simulink model "distribution"  (R2015a)
settings: Solver=ode45  StartTime=0  StopTime=1000  RelTol=1e-3
libraries: simulink x1
(part 1 of 2)
settings Model: Creator=tzimi  LastModifiedBy=Tzimisce

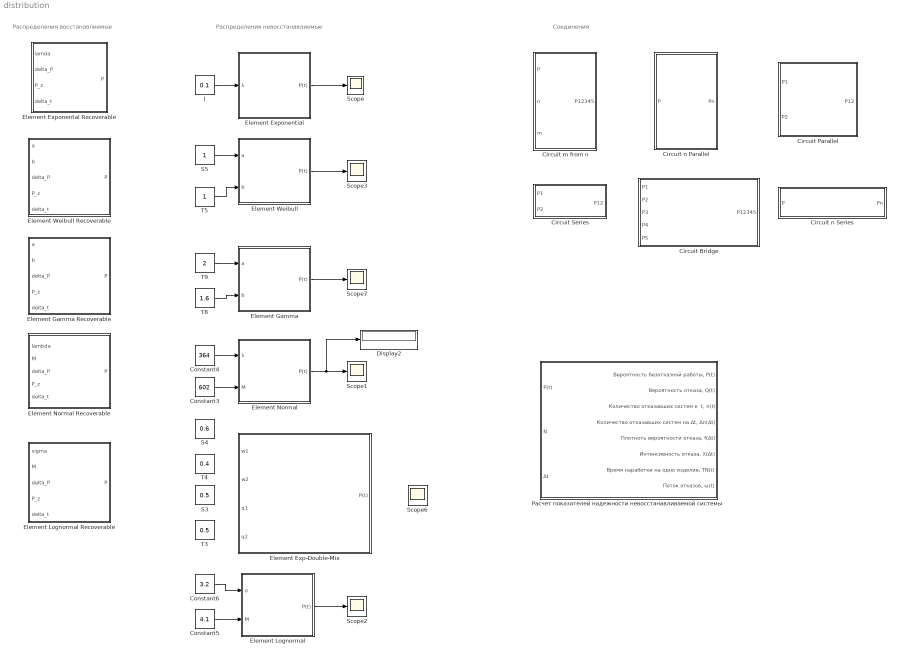
== system distribution ==
  note: Соединения
  note: Распределения невосстанавлиемые
  note: Распределения восстанавлиемые
  Constant3 : Constant  Value=602
  Constant4 : Constant  Value=364
  Constant5 : Constant  Value=4.1
  Constant6 : Constant  Value=3.2
  Display2 : Display
  Element Gamma : Subsystem  mask(Element Gamma){}
      mask help:
      | <p>Возвращает вероятность безотказной работы невосстанавливаемого элемента
      |  по гамма-распределению.</p>
      | <p>Гамма-распределение является результатом смешения большого
      | числа потоков имеющих экспоненциальное распределение.</p>
      | <p>Гамма-распределение используется при оценке надежности объектов, причиной
      | отказа которых является коррозия, вибрация, статическая нагрузка,
      | ошибка персонала и т.д.</p>
      mask Help:
      | <p>Возвращает вероятность безотказной работы невосстанавливаемого элемента
      |  по гамма-распределению.</p>
      | <p>Гамма-распределение используется при оценке надежности объектов, причиной
      | отказа которых является коррозия, вибрация, статическая нагрузка,
      | ошибка персонала и т.д.</p>
      | <p>Входные параметры:</p>
      | <p>a - параметр места гамма-распределения,</p>
      | <p>b - параметр формы гамма-распределения.</p>
      | <p>Выходной параметр P(t) - вероятность безотказной работы элемента.</p>
      mask Display:
      | image('images/png/gamma.png')
      | port_label('input', 1, 'a')
      | port_label('input', 2, 'b')
      | port_label('output', 1, 'P(t)')
  Element Gamma Recoverable : Subsystem  mask(Element Gamma Recoverable){}
      mask help:
      | <p>Возвращает вероятность безотказной работы восстанавливаемого элемента
      | по гамма-распределению.</p>
      | <p>Гамма-распределение является результатом смешения большого
      | числа потоков имеющих экспоненциальное распределение.</p>
      | <p>Гамма-распределение используется при оценке надежности объектов, причиной
      | отказа которых является коррозия, вибрация, статическая нагрузка,
      | ошибка персонала и т.д.</p>
      mask Help:
      | <p>Возвращает вероятность безотказной работы восстанавливаемого элемента
      |  по гамма-распределению.</p>
      | <p>Гамма-распределение используется при оценке надежности объектов, причиной
      | отказа которых является коррозия, вибрация, статическая нагрузка,
      | ошибка персонала и т.д.</p>
      | <p>Входные параметры:</p>
      | <p>a - параметр места гамма-распределения,</p>
      | <p>b - параметр формы гамма-распределения,</p>
      | <p>ΔP - на сколько снижается вероятность безотказной работы после
      | восстановления элемента,</p>
      | <p>Pз - заданная вероятность, после которой проводится восстановление элемента,</p>
      | <p>Δt - время восстановления элемента.</p>
      | <p>Выходной параметр P(t) - вероятность безотказной работы элемента.</p>
      mask Display:
      | image('images/gamma_req.png')
      | port_label('input', 1, 'a')
      | port_label('input', 2, 'b')
      | port_label('input', 3, 'ΔP')
      | port_label('input', 4, 'Pз')
      | port_label('input', 5, 'Δt')
      | port_label('output', 1, 'P(t)')
  Element Exp-Double-Mix : Subsystem  mask(Element Exp-Double-Mix){}
      mask help:
      | <p>Возвращает вероятность безотказной работы двух элементов по экспоненциальному
      | закону распределения.</p>
      | <p>При оценке надежности смеси двух экспоненциальных распределений результатом
      | является поток отказов-восстановлений объектов, составленный из потока отказов
      | с параметром ω1 и потока восстановлений с параметром ω2.</p>
      | <p>Если эти потоки в общем случае не равнодолевые (то есть, не каждый отказ
      | сопровождается полным восстановлением объекта), то необходимо учитывать и
      | доли потоков: q1 и q2 (q1 + q2 = 1).</p>
      mask Help:
      | <p>Возвращает вероятность безотказной работы двух элементов по экспоненциальному
      | закону распределения.</p>
      | <p>Входные параметры:</p>
      | <p>ω1 - поток отказов,</p>
      | <p>ω2 - поток восстановлений,</p>
      | <p>q1 - доля потока отказов,</p>
      | <p>q2 - доля потока восстановления.</p>
      | <p>Выходной параметр P(t) - вероятность безотказной работы элемента.</p>
      mask Display:
      | image('images/png/exp.png')
      | port_label('input', 1, 'ω1')
      | port_label('input', 2, 'ω2')
      | port_label('input', 3, 'q1')
      | port_label('input', 4, 'q2')
      | port_label('output', 1, 'P(t)')
  "Element Exponental Recoverable " : Subsystem  mask(Element Exponental Recoverable){}
      mask help:
      | <p>Возвращает вероятность безотказной работы восстанавливаемого элемента
      | по экспоненциальному закону распределения.</p>
      | <p>Экспоненциальное (или показательное) распределение — абсолютно непрерывное
      | распределение, моделирующее время между двумя последовательными свершениями
      | одного и того же события.</p>
      | <p>Экспоненциальное распределение используют при оценке надежности сложных
      | технических систем, не подверженных износу и старению и в случаях, когда
      | отказы объектов имеют случайный характер.</p>
      mask Help:
      | <p>Возвращает вероятность безотказной работы восстанавливаемого элемента по экспоненциальному
      | закону распределения.</p>
      | <p>Экспоненциальное распределение используют при оценке надежности сложных
      | технических систем, не подверженных износу и старению и в случаях, когда
      | отказы объектов имеют случайный характер.</p>
      | <p>Входные параметры:</p>
      | <p>λ - интенсивность событий в рассматриваемом потоке,</p>
      | <p>ΔP - на сколько снижается вероятность безотказной работы после
      | восстановления элемента,</p>
      | <p>Pз - заданная вероятность, после которой проводится восстановление элемента,</p>
      | <p>Δt - время восстановления элемента.</p>
      | <p>Выходной параметр P(t) - вероятность безотказной работы элемента.</p>
      mask Display:
      | image('images/exp_req.png')
      | port_label('input', 1, 'λ')
      | port_label('input', 2, 'ΔP')
      | port_label('input', 3, 'Pз')
      | port_label('input', 4, 'Δt')
      | port_label('output', 1, 'P(t)')
  Element Exponential : Subsystem  mask(Element Exponential){}
      mask help:
      | <p>Возвращает вероятность безотказной работы невосстанавливаемого элемента
      | по экспоненциальному закону распределения.</p>
      | <p>Экспоненциальное (или показательное) распределение — абсолютно непрерывное
      | распределение, моделирующее время между двумя последовательными свершениями
      | одного и того же события.</p>
      | <p>Экспоненциальное распределение используют при оценке надежности сложных
      | технических систем, не подверженных износу и старению и в случаях, когда
      | отказы объектов имеют случайный характер.</p>
      mask Help:
      | <p>Возвращает вероятность безотказной работы невосстанавливаемого элемента по экспоненциальному
      | закону распределения.</p>
      | <p>Экспоненциальное распределение используют при оценке надежности сложных
      | технических систем, не подверженных износу и старению и в случаях, когда
      | отказы объектов имеют случайный характер.</p>
      | <p>Входной параметр λ - интенсивность событий в рассматриваемом потоке.</p>
      | <p>Выходной параметр P(t) - вероятность безотказной работы элемента.</p>
      mask Display:
      | image('images/png/exp.png')
      | port_label('input', 1, 'λ')
      | port_label('output', 1, 'P(t)')
  "Element Lognormal " : Subsystem  mask(Element Lognormal){}
      mask help:
      | <p>Возвращает вероятность безотказной работы невосстанавливаемого элемента
      | по логнормальному закону распределения.</p>
      | <p>Логнормальное распределение — это двухпараметрическое семейство
      | абсолютно непрерывных распределений. Если случайная величина имеет
      | логнормальное распределение, то её логарифм имеет нормальное распределение.</p>
      | <p>Логнормальное распределение обычно используют при оценке надежности
      | элементов, для которых основной причиной отказа является усталость,
      | обусловленная периодическим многоцикловым (вибрационным) нагружением.</p>
      mask Help:
      | <p>Возвращает вероятность безотказной работы невосстанавливаемого элемента
      | по логнормальному закону распределения.</p>
      | <p>Логнормальное распределение обычно используют при оценке надежности
      | элементов, для которых основной причиной отказа является усталость,
      | обусловленная периодическим многоцикловым (вибрационным) нагружением.</p>
      | <p>Входные параметры:</p>
      | <p>σ - среднее квадратическое отклонение наработки до отказа,</p>
      | <p>М - математическое ожидание наработки до отказа.</p>
      | <p>Выходной параметр P(t) - вероятность безотказной работы элемента.</p>
      mask Display:
      | image('images/png/log_normal.png')
      | port_label('input', 1, 'σ')
      | port_label('input', 2, 'M')
      | port_label('output', 1, 'P(t)')
  Element Lognormal Recoverable : Subsystem  mask(Element Lognormal Recoverable){}
      mask help:
      | <p>Возвращает вероятность безотказной работы восстанавливаемого элемента
      | по логнормальному закону распределения.</p>
      | <p>Логнормальное распределение — это двухпараметрическое семейство
      | абсолютно непрерывных распределений. Если случайная величина имеет
      | логнормальное распределение, то её логарифм имеет нормальное распределение.</p>
      | <p>Логнормальное распределение обычно используют при оценке надежности
      | элементов, для которых основной причиной отказа является усталость,
      | обусловленная периодическим многоцикловым (вибрационным) нагружением.</p>
      mask Help:
      | <p>Возвращает вероятность безотказной работы восстанавливаемого элемента
      | по логнормальному закону распределения.</p>
      | <p>Логнормальное распределение обычно используют при оценке надежности
      | элементов, для которых основной причиной отказа является усталость,
      | обусловленная периодическим многоцикловым (вибрационным) нагружением.</p>
      | <p>Входные параметры:</p>
      | <p>σ - среднее квадратическое отклонение наработки до отказа,</p>
      | <p>М - математическое ожидание наработки до отказа,</p>
      | <p>ΔP - на сколько снижается вероятность безотказной работы после
      | восстановления элемента,</p>
      | <p>Pз - заданная вероятность, после которой проводится восстановление элемента,</p>
      | <p>Δt - время восстановления элемента.</p>
      | <p>Выходной параметр P(t) - вероятность безотказной работы элемента.</p>
      mask Display:
      | image('images/log_normal_req.png')
      | port_label('input', 1, 'σ')
      | port_label('input', 2, 'M')
      | port_label('input', 3, 'ΔP')
      | port_label('input', 4, 'Pз')
      | port_label('input', 5, 'Δt')
      | port_label('output', 1, 'P(t)')
  Element Normal : Subsystem  mask(Element Normal){}
      mask help:
      | <p>Возвращает вероятность безотказной работы невосстанавливаемого
      | элемента по нормальному закону распределения.</p>
      | <p>Нормальное распределение, также называемое распределением Гаусса или
      | Гаусса — Лапласа — распределение вероятностей, которое в одномерном
      | случае задаётся функцией плотности вероятности, совпадающей с функцией
      | Гаусса.</p>
      | <p>Нормальное распределение обычно используют при оценке надежности объектов,
      | основной причиной отказа которых является износ.</p>
      mask Help:
      | <p>Возвращает вероятность безотказной работы невосстанавливаемого
      | элемента по нормальному закону распределения.</p>
      | <p>Нормальное распределение обычно используют при оценке надежности объектов,
      | основной причиной отказа которых является износ.</p>
      | <p>Входные параметры:</p>
      | <p>λ - среднее квадратическое отклонение наработки до отказа,</p>
      | <p>М - математическое ожидание наработки до отказа.</p>
      | <p>Выходной параметр P(t) - вероятность безотказной работы элемента.</p>
      mask Display:
      | image('images/png/normal_nogrid.png')
      | port_label('input', 1, 'λ')
      | port_label('input', 2, 'M')
      | port_label('output', 1, 'P(t)')
  Element Normal Recoverable : Subsystem  mask(Element Normal Recoverable){}
      mask help:
      | <p>Возвращает вероятность безотказной работы восстанавливаемого
      | элемента по нормальному закону распределения.</p>
      | <p>Нормальное распределение, также называемое распределением Гаусса или
      | Гаусса — Лапласа — распределение вероятностей, которое в одномерном
      | случае задаётся функцией плотности вероятности, совпадающей с функцией
      | Гаусса.</p>
      | <p>Нормальное распределение обычно используют при оценке надежности объектов,
      | основной причиной отказа которых является износ.</p>
      mask Help:
      | <p>Возвращает вероятность безотказной работы восстанавливаемого
      | элемента по нормальному закону распределения.</p>
      | <p>Нормальное распределение обычно используют при оценке надежности объектов,
      | основной причиной отказа которых является износ.</p>
      | <p>Входные параметры:</p>
      | <p>λ - среднее квадратическое отклонение наработки до отказа,</p>
      | <p>М - математическое ожидание наработки до отказа,</p>
      | <p>ΔP - на сколько снижается вероятность безотказной работы после
      | восстановления элемента,</p>
      | <p>Pз - заданная вероятность, после которой проводится восстановление элемента,</p>
      | <p>Δt - время восстановления элемента.</p>
      | <p>Выходной параметр P(t) - вероятность безотказной работы элемента.</p>
      mask Display:
      | image('images/normal_nogrid_req.png')
      | port_label('input', 1, 'λ')
      | port_label('input', 2, 'M')
      | port_label('input', 3, 'ΔP')
      | port_label('input', 4, 'Pз')
      | port_label('input', 5, 'Δt')
      | port_label('output', 1, 'P(t)')
  Element Weibull : Subsystem  mask(Element Weibull){}
      mask help:
      | <p>Возвращает вероятность безотказной работы невосстанавливаемого элемента по закону
      | распределения Вейбулла .</p>
      | <p>Распределение Вейбулла — это распределение случайной величины с
      | использованием экспоненты в функциях распределения.</p>
      | <p>Распределение Вейбулла используют для описания закономерностей отказов
      | под действием износа и старения, отказов последовательно соединенных и
      | дублированных элементов. Особенно часто распределение Вейбулла применяют
      | тогда, когда поток отказов не стационарен и интенсивность отказов меняется
      | с течением времени.</p>
      mask Help:
      | <p>Возвращает вероятность безотказной работы невосстанавливаемого элемента по закону
      | распределения Вейбулла .</p>
      | <p>Распределение Вейбулла используют для описания закономерностей отказов
      | под действием износа и старения, отказов последовательно соединенных и
      | дублированных элементов. Особенно часто распределение Вейбулла применяют
      | тогда, когда поток отказов не стационарен и интенсивность отказов меняется
      | с течением времени.</p>
      | <p>Входные параметры:</p>
      | <p>а - параметр места распределения Вейбулла,</p>
      | <p>b - параметр формы распределения Вейбулла.</p>
      | <p>Выходной параметр P(t) - вероятность безотказной работы элемента.</p>
      mask Display:
      | image('images/png/weibull.png')
      | port_label('input', 1, 'a')
      | port_label('input', 2, 'b')
      | port_label('output', 1, 'P(t)')
  Element Weibull Recoverable : Subsystem  mask(Element Weibull Recoverable){}
      mask help:
      | <p>Возвращает вероятность безотказной работы восстанавливаемого элемента по закону
      | распределения Вейбулла .</p>
      | <p>Распределение Вейбулла — это распределение случайной величины с
      | использованием экспоненты в функциях распределения.</p>
      | <p>Распределение Вейбулла используют для описания закономерностей отказов
      | под действием износа и старения, отказов последовательно соединенных и
      | дублированных элементов. Особенно часто распределение Вейбулла применяют
      | тогда, когда поток отказов не стационарен и интенсивность отказов меняется
      | с течением времени.</p>
      mask Help:
      | <p>Возвращает вероятность безотказной работы восстанавливаемого элемента по закону
      | распределения Вейбулла.</p>
      | <p>Распределение Вейбулла используют для описания закономерностей отказов
      | под действием износа и старения, отказов последовательно соединенных и
      | дублированных элементов. Особенно часто распределение Вейбулла применяют
      | тогда, когда поток отказов не стационарен и интенсивность отказов меняется
      | с течением времени.</p>
      | <p>Входные параметры:</p>
      | <p>а - параметр места распределения Вейбулла,</p>
      | <p>b - параметр формы распределения Вейбулла,</p>
      | <p>ΔP - на сколько снижается вероятность безотказной работы после
      | восстановления элемента,</p>
      | <p>Pз - заданная вероятность, после которой проводится восстановление элемента,</p>
      | <p>Δt - время восстановления элемента.</p>
      | <p>Выходной параметр P(t) - вероятность безотказной работы элемента.</p>
      mask Display:
      | image('images/weibull_req.png')
      | port_label('input', 1, 'a')
      | port_label('input', 2, 'b')
      | port_label('input', 3, 'ΔP')
      | port_label('input', 4, 'Pз')
      | port_label('input', 5, 'Δt')
      | port_label('output', 1, 'P(t)')
  S3 : Constant  Value=0.5
  S4 : Constant  Value=0.6
  S5 : Constant
  Scope{,1..3,6..7} (6 alike) : Scope
      Scope settings: YMin=-0.12495  YMax=1.12499
      Scope1 settings: TimeRange=20  YMin=-0.97508  YMax=0.10834
      Scope2 settings: YMin=-2.66158  YMax=1.40684  SaveName=ScopeData2
      Scope3 settings: TimeRange=20  YMin=-0.125  YMax=1.125  SaveName=ScopeData3
      Scope6 settings: YMin=-0.12477  YMax=1.12497  SaveName=ScopeData6
      Scope7 settings: TimeRange=20  YMin=-0.12409  YMax=1.11677  SaveName=ScopeData7
  T3 : Constant  Value=0.5
  T4 : Constant  Value=0.4
  T5 : Constant
  T8 : Constant  Value=1.6
  T9 : Constant  Value=2
  l : Constant  Value=0.1
  Расчет показателей надежности невосстанавливаемой системы : Subsystem  mask(Calculation of reliability indicators of an unrecoverable system.){}
      mask help:
      | <p>Расчет показателей надежности невосстанавливаемой системы.</p>
      | <p>Возвращает показатели надежности невосстанавливаемой системы.</p>
      | <p>Показателями надежности называются количественные характеристики одного
      | или нескольких свойств, составляющих надежность системы.</p>
      mask Help:
      | <p>Возвращает показатели надежности невосстанавливаемой системы.</p>
      | <p>Показателями надежности называются количественные характеристики одного
      | или нескольких свойств, составляющих надежность системы.</p>
      | <p>Входные параметры:</p>
      | <p>P(t)- вероятность безотказной работы элемента,</p>
      | <p>N - количество элементов,</p>
      | <p>Δt - шаг времени.</p>
      | <p>Выходной параметры:</p>
      | <p>P(t)- вероятность безотказной работы элемента,</p>
      | <p>Q(t) - вероятность отказа элемента,</p>
      | <p>n(t) - количество отказавших систем ко времени t,</p>
      | <p>Δn(Δt) - количество отказавших систем на момент времени Δt,</p>
      | <p>f(Δt) - плотноть вероятности отказа,</p>
      | <p>λ(Δt) - интенсивность отказа,</p>
      | <p>TN(t) - время наработки на одно изделие,</p>
      | <p>ω(t) - поток отказов.</p>
      mask Display:
      | port_label('input', 1, 'P(t)')
      | port_label('input', 2, 'N')
      | port_label('input', 3, 'Δt')
      | port_label('output', 1, 'P(t)')
      | port_label('output', 2, 'Q(t)')
      | port_label('output', 3, 'n(t)')
      | port_label('output', 4, 'Δn(Δt)')
      | port_label('output', 5, 'f(Δt)')
      | port_label('output', 6, 'λ(Δt)')
      | port_label('output', 7, 'TN(t)')
      | port_label('output', 8, 'ω(t)')
  Сircuit Bridge : Subsystem  mask(Сircuit Bridge){}
      mask help:
      | <p>Возвращает вероятность безотказной работы пяти элементов, соединенных
      | мостиковой схемой.</p>
      | <p>Мостиковой схемой называется параллельное соединение последовательных
      | цепочек элементов с диагональными элементами, включенными между узлами
      | различных параллельных ветвей.</p>
      | <p>Работоспособность мостиковой схемы зависит не только от количества отказавших
      | элементов, но и от их положения в структурной схеме.</p>
      mask Help:
      | <p>Возвращает вероятность безотказной работы пяти элементов, соединенных
      | мостиковой схемой.</p>
      | <p>Работоспособность мостиковой схемы зависит не только от количества отказавших
      | элементов, но и от их положения в структурной схеме. При одновременном отказе
      | элементов 1 и 4, или 2 и 5, или 2, 3 и 4 и т.д. схема окажется неработоспособной.
      | Но отказ элементов 1 и 5, или 2 и 4, или 1, 3 и 4, или 2, 3 и 5 к отказу
      | системы не приводит.</p>
      | <p>Входные параметры:</p>
      | <p>P1 - вероятность безотказной работы первого элемента,</p>
      | <p>P2 - вероятность безотказной работы второго элемента,</p>
      | <p>P3 - вероятность безотказной работы третьего элемента,</p>
      | <p>P4 - вероятность безотказной работы четвертого элемента,</p>
      | <p>P5 - вероятность безотказной работы пятого элемента.</p>
      | <p>Выходной параметр P(t) - вероятность безотказной работы всех элементов.</p>
      mask Display:
      | image('images\png\bridge.png')
      | port_label('input', 1, 'P1')
      | port_label('input', 2, 'P2')
      | port_label('input', 3, 'P3')
      | port_label('input', 4, 'P4')
      | port_label('input', 5, 'P5')
      | port_label('output', 1, 'P')
  Сircuit Parallel : Subsystem  mask(Сircuit Parallel){}
      mask help:
      | <p>Возвращает вероятность безотказной работы двух параллельно соединенных
      | элементов.</p>
      | <p>В системе с параллельной структурой отказ системы в целом происходит только
      | при отказе всех элементов.</p>
      mask Help:
      | <p>Возвращает вероятность безотказной работы двух параллельно соединенных
      | элементов.</p>
      | <p>Входные параметры:</p>
      | <p>P1 - вероятность безотказной работы первого элемента,</p>
      | <p>P2 - вероятность безотказной работы второго элемента.</p>
      | <p>Выходной параметр P12 - вероятность безотказной работы двух параллельно
      | соединенных элементов.</p>
      mask Display:
      | image('images/png/parallel2.png')
      | port_label('input', 1, 'P1')
      | port_label('input', 2, 'P2')
      | port_label('output', 1, 'P12')
  Сircuit Series : Subsystem  mask(Сircuit Series){}
      mask help:
      | <p>Возвращает вероятность безотказной работы двух последовательно соединенных
      | элементов.</p>
      | <p>В системе с последовательной структурой отказ любого компонента приводит
      | к отказу системы в целом.</p>
      mask Help:
      | <p>Возвращает вероятность безотказной работы двух последовательно соединенных
      | элементов.</p>
      | <p>Входные параметры:</p>
      | <p>P1 - вероятность безотказной работы первого элемента,</p>
      | <p>P2 - вероятность безотказной работы второго элемента.</p>
      | <p>Выходной параметр P12 - вероятность безотказной работы двух последовательно
      | соединенных элементов.</p>
      mask Display:
      | image('images/png/series2.png')
      | port_label('input', 1, 'P1')
      | port_label('input', 2, 'P2')
      | port_label('output', 1, 'P12')
  Сircuit m from n : Subsystem  mask(Сircuit m from n){}
      mask help:
      | <p>Возвращает вероятность того, что в системе, состоящей из n одинаковых
      | (равнонадежных) элементов, безотказно работают ровно m элементов.</p>
      | <p>Система типа “m из n” это вариант системы с параллельным соединением
      | элементов, отказ которой произойдет, если из n элементов, соединенных
      | параллельно, работоспособными окажутся менее m элементов (m < n).</p>
      mask Help:
      | <p>Возвращает вероятность того, что в системе, состоящей из n одинаковых
      | (равнонадежных) элементов, безотказно работают ровно k элементов.</p>
      | <p>Входные параметры:</p>
      | <p>P - вероятность безотказной работы n равнонадежных элементов,</p>
      | <p>n - количество элементов в системе,</p>
      | <p>m - количество элементов, необходимых для работоспособности системы.</p>
      | <p>Выходной параметр Pm - вероятность безотказной работы m элементов системы.</p>
      mask Display:
      | image('images\png\mn.png')
      | port_label('input', 1, 'P')
      | port_label('input', 2, 'n')
      | port_label('input', 3, 'm')
      | port_label('output', 1, 'Pm')
  Сircuit n Parallel : Subsystem  mask(Сircuit n Parallel){}
      mask help:
      | <p>Возвращает вероятность безотказной работы n параллельно соединенных
      | элементов.</p>
      | <p>В системе с параллельной структурой отказ системы в целом происходит только
      | при отказе всех элементов.</p>
      mask Help:
      | <p>Возвращает вероятность безотказной работы n параллельно соединенных
      | элементов.</p>
      | <p>Входной параметр P - массив вероятностей безотказной работы элементов.</p>
      | <p>Выходной параметр Pт - вероятность безотказной работы n параллельно
      | соединенных элементов.</p>
      mask Display:
      | image('images\png\parallel.png')
      | port_label('input', 1, 'P')
      | port_label('output', 1, 'Pn')
  Сircuit n Series : Subsystem  mask(Сircuit n Series){}
      mask help:
      | <p>Возвращает вероятность безотказной работы n последовательно соединенных
      | элементов.</p>
      | <p>В системе с последовательной структурой отказ любого компонента приводит
      | к отказу системы в целом.</p>
      mask Help:
      | <p>Возвращает вероятность безотказной работы n последовательно соединенных
      | элементов.</p>
      | <p>Входной параметр P - массив вероятностей безотказной работы n элементов.</p>
      | <p>Выходной параметр Pn - вероятность безотказной работы n последовательно
      | соединенных элементов.</p>
      mask Display:
      | image('images\png\series.png')
      | port_label('input', 1, 'P')
      | port_label('output', 1, 'Pn')
  wires:
  Constant4/1 -> Element Normal/1("λ ")
  Constant3/1 -> Element Normal/2("M ")
  Element Normal/1(P(t)) -> Display2/1, Scope1/1
  T9/1 -> Element Gamma/1(a)
  T8/1 -> Element Gamma/2(b)
  Element Gamma/1(P(t)) -> Scope7/1
  Element Exponential/1(P(t)) -> Scope/1
  Element Weibull/1(P(t)) -> Scope3/1
  l/1 -> Element Exponential/1("λ ")
  S5/1 -> Element Weibull/1("a ")
  T5/1 -> Element Weibull/2("b ")
  Constant6/1 -> "Element Lognormal "/1("σ ")
  Constant5/1 -> "Element Lognormal "/2("M ")
  "Element Lognormal "/1(P(t)) -> Scope2/1

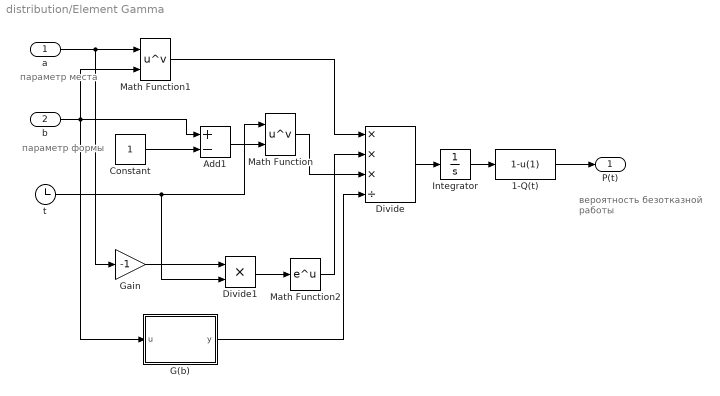
== system distribution/Element Gamma ==
  note: параметр
      | формы
  note: параметр
      | места
  note: вероятность
      | безотказной
      | работы
  a : Inport
  b : Inport  Port=2
  1-Q(t) : Fcn  Expr=1-u(1)
  Add1 : Sum  Inputs=+-
  Constant : Constant
  Divide : Product  Inputs=***/
  Divide1 : Product  Inputs=**
  G(b) : MATLAB Function  TreatAsAtomicUnit=on
  Gain : Gain  Gain=-1
  Integrator : Integrator
  Math Function : Math  Operator=pow  SaturateOnIntegerOverflow=on
  Math Function1 : Math  Operator=pow  SaturateOnIntegerOverflow=on
  Math Function2 : Math  SaturateOnIntegerOverflow=on
  t : Clock
  P(t) : Outport
  wires:
  b/1 -> Add1/1, Math Function1/2, G(b)/1(u)
  Add1/1 -> Math Function/2
  a/1 -> Math Function1/1, Gain/1
  Math Function1/1 -> Divide/1
  Gain/1 -> Divide1/1
  Divide1/1 -> Math Function2/1
  Math Function2/1 -> Divide/2
  Constant/1 -> Add1/2
  1-Q(t)/1 -> P(t)/1
  Divide/1 -> Integrator/1
  Math Function/1 -> Divide/3
  Integrator/1 -> 1-Q(t)/1
  t/1 -> Divide1/2, Math Function/1
  G(b)/1(y) -> Divide/4

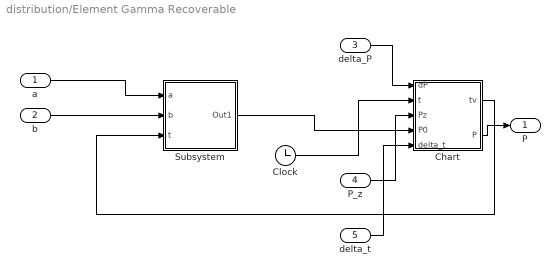
== system distribution/Element Gamma Recoverable ==
  a : Inport
  b : Inport  Port=2
  delta_P : Inport  Port=3
  P_z : Inport  Port=4
  delta_t : Inport  Port=5
  Chart : Stateflow chart  TreatAsAtomicUnit=on
  Clock : Clock
  Subsystem : Subsystem
  P : Outport
  wires:
  Subsystem/1(Out1) -> Chart/4(P0)
  Chart/2(P) -> P/1
  P_z/1 -> Chart/3(Pz)
  delta_P/1 -> Chart/1(dP)
  Clock/1 -> Chart/2(t)
  a/1 -> Subsystem/1(a)
  b/1 -> Subsystem/2(b)
  Chart/1(tv) -> Subsystem/3(t)
  delta_t/1 -> Chart/5(delta_t)

== system distribution/Element Exp-Double-Mix ==
  note: Доля потока
      | восстановления
  note: Доля потока отказов
  note: Параметр поток
      | восстановлений
  note: Параметр поток отказов
  note: вероятность
      | безотказной
      | работы
  "w1 " : Inport
  "w2 " : Inport  Port=2
  "q1 " : Inport  Port=3
  "q2 " : Inport  Port=4
  Mux : Mux  Inputs=5
  f(t) : Fcn  Expr=(u(3)*u(2)*exp((-1)*u(1)*u(5))+u(4)*u(1)*exp((-1)*u(2)*u(5)))/(u(1)*u(4)+u(2)*u(3))
  t : Clock
  P(t) : Outport
  wires:
  "q1 "/1 -> Mux/3
  t/1 -> Mux/5
  "w1 "/1 -> Mux/1
  f(t)/1 -> P(t)/1
  "w2 "/1 -> Mux/2
  "q2 "/1 -> Mux/4
  Mux/1 -> f(t)/1

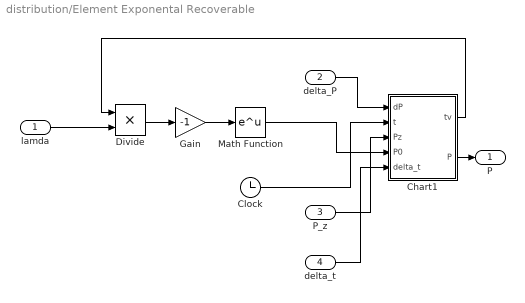
== system distribution/Element Exponental Recoverable  ==
  lamda : Inport
  delta_P : Inport  Port=2
  P_z : Inport  Port=3
  delta_t : Inport  Port=4
  Chart1 : Stateflow chart  TreatAsAtomicUnit=on
  Clock : Clock
  Divide : Product  Inputs=**
  Gain : Gain  Gain=-1
  Math Function : Math  SaturateOnIntegerOverflow=on
  P : Outport
  wires:
  Chart1/2(P) -> P/1
  P_z/1 -> Chart1/3(Pz)
  Math Function/1 -> Chart1/4(P0)
  delta_P/1 -> Chart1/1(dP)
  Chart1/1(tv) -> Divide/1
  Clock/1 -> Chart1/2(t)
  lamda/1 -> Divide/2
  Gain/1 -> Math Function/1
  Divide/1 -> Gain/1
  delta_t/1 -> Chart1/5(delta_t)

== system distribution/Element Exponential ==
  note: интенсивность событий
      | в рассматриваемом потоке
  note: вероятность
      | безотказной
      | работы
  "λ " : Inport
  Divide : Product  Inputs=**
  Gain : Gain  Gain=-1
  Math Function : Math  SaturateOnIntegerOverflow=on
  t : Clock
  P(t) : Outport
  wires:
  Divide/1 -> Gain/1
  t/1 -> Divide/1
  Gain/1 -> Math Function/1
  Math Function/1 -> P(t)/1
  "λ "/1 -> Divide/2

== system distribution/Element Lognormal  ==
  note: среднее квадратическое
      | отклонение наработки
      | до отказа
  note: математическое ожидание
      | наработки до отказа
  note: вероятность
      | безотказной
      | работы
  "σ " : Inport
  "M " : Inport  Port=2
  Fcn1 : Fcn  Expr=1-u(1)
  MATLAB Function : MATLAB Function  TreatAsAtomicUnit=on
  t : Clock
  P(t) : Outport
  wires:
  MATLAB Function/1(y) -> Fcn1/1
  Fcn1/1 -> P(t)/1
  t/1 -> MATLAB Function/1(t)
  "σ "/1 -> MATLAB Function/2(sigma)
  "M "/1 -> MATLAB Function/3(M)

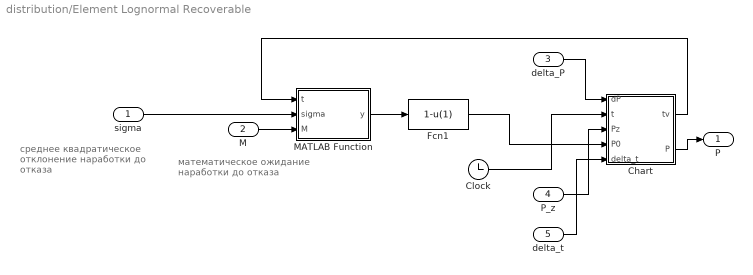
== system distribution/Element Lognormal Recoverable ==
  note: среднее квадратическое
      | отклонение наработки
      | до отказа
  note: математическое ожидание
      | наработки до отказа
  "sigma " : Inport
  "M " : Inport  Port=2
  delta_P : Inport  Port=3
  P_z : Inport  Port=4
  delta_t : Inport  Port=5
  Chart : Stateflow chart  TreatAsAtomicUnit=on
  Clock : Clock
  Fcn1 : Fcn  Expr=1-u(1)
  MATLAB Function : MATLAB Function  TreatAsAtomicUnit=on
  P : Outport
  wires:
  Chart/2(P) -> P/1
  P_z/1 -> Chart/3(Pz)
  delta_P/1 -> Chart/1(dP)
  Clock/1 -> Chart/2(t)
  MATLAB Function/1(y) -> Fcn1/1
  Chart/1(tv) -> MATLAB Function/1(t)
  "sigma "/1 -> MATLAB Function/2(sigma)
  "M "/1 -> MATLAB Function/3(M)
  Fcn1/1 -> Chart/4(P0)
  delta_t/1 -> Chart/5(delta_t)

== system distribution/Element Normal ==
  note: вероятность
      | безотказной
      | работы
  note: математическое ожидание
      | наработки до отказа
  note: среднее квадратическое
      | отклонение наработки
      | до отказа
  "λ " : Inport
  "M " : Inport  Port=2
  1-Q(t)1 : Fcn  Expr=1-u(1)
  MATLAB Function : MATLAB Function  TreatAsAtomicUnit=on
  t : Clock
  P(t) : Outport
  wires:
  MATLAB Function/1(y) -> 1-Q(t)1/1
  "λ "/1 -> MATLAB Function/2(sigma)
  1-Q(t)1/1 -> P(t)/1
  t/1 -> MATLAB Function/1(t)
  "M "/1 -> MATLAB Function/3(M)

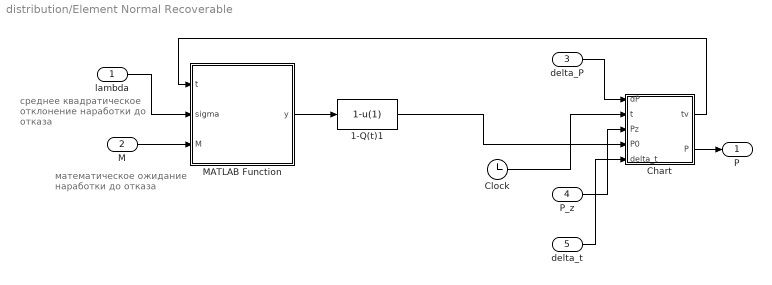
== system distribution/Element Normal Recoverable ==
  note: математическое ожидание
      | наработки до отказа
  note: среднее квадратическое
      | отклонение наработки
      | до отказа
  "lambda " : Inport
  "M " : Inport  Port=2
  delta_P : Inport  Port=3
  P_z : Inport  Port=4
  delta_t : Inport  Port=5
  1-Q(t)1 : Fcn  Expr=1-u(1)
  Chart : Stateflow chart  TreatAsAtomicUnit=on
  Clock : Clock
  MATLAB Function : MATLAB Function  TreatAsAtomicUnit=on
  P : Outport
  wires:
  Clock/1 -> Chart/2(t)
  delta_P/1 -> Chart/1(dP)
  P_z/1 -> Chart/3(Pz)
  Chart/2(P) -> P/1
  1-Q(t)1/1 -> Chart/4(P0)
  MATLAB Function/1(y) -> 1-Q(t)1/1
  "lambda "/1 -> MATLAB Function/2(sigma)
  "M "/1 -> MATLAB Function/3(M)
  Chart/1(tv) -> MATLAB Function/1(t)
  delta_t/1 -> Chart/5(delta_t)

== system distribution/Element Weibull ==
  note: параметр формы
  note: параметр места
  note: вероятность
      | безотказной
      | работы
  "a " : Inport
  "b " : Inport  Port=2
  Mux : Mux  Inputs=3
  f(t) : Fcn  Expr=exp((-1)*u(3)^(u(2))*u(1)^(-1))
  задаваемая наработка : Clock
  P(t) : Outport
  wires:
  "a "/1 -> Mux/1
  f(t)/1 -> P(t)/1
  Mux/1 -> f(t)/1
  задаваемая наработка/1 -> Mux/3
  "b "/1 -> Mux/2

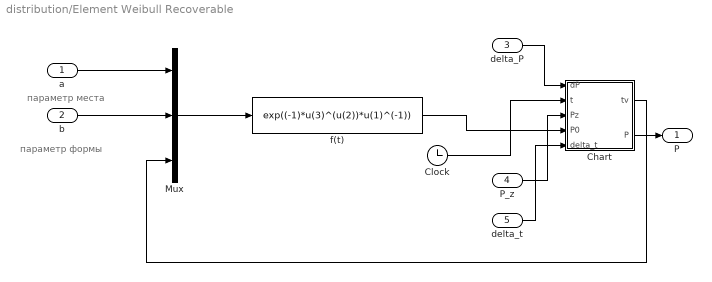
== system distribution/Element Weibull Recoverable ==
  note: параметр формы
  note: параметр места
  "a " : Inport
  "b " : Inport  Port=2
  delta_P : Inport  Port=3
  P_z : Inport  Port=4
  delta_t : Inport  Port=5
  Chart : Stateflow chart  TreatAsAtomicUnit=on
  Clock : Clock
  Mux : Mux  Inputs=3
  f(t) : Fcn  Expr=exp((-1)*u(3)^(u(2))*u(1)^(-1))
  P : Outport
  wires:
  Clock/1 -> Chart/2(t)
  delta_P/1 -> Chart/1(dP)
  P_z/1 -> Chart/3(Pz)
  Chart/2(P) -> P/1
  "a "/1 -> Mux/1
  f(t)/1 -> Chart/4(P0)
  Mux/1 -> f(t)/1
  Chart/1(tv) -> Mux/3
  "b "/1 -> Mux/2
  delta_t/1 -> Chart/5(delta_t)

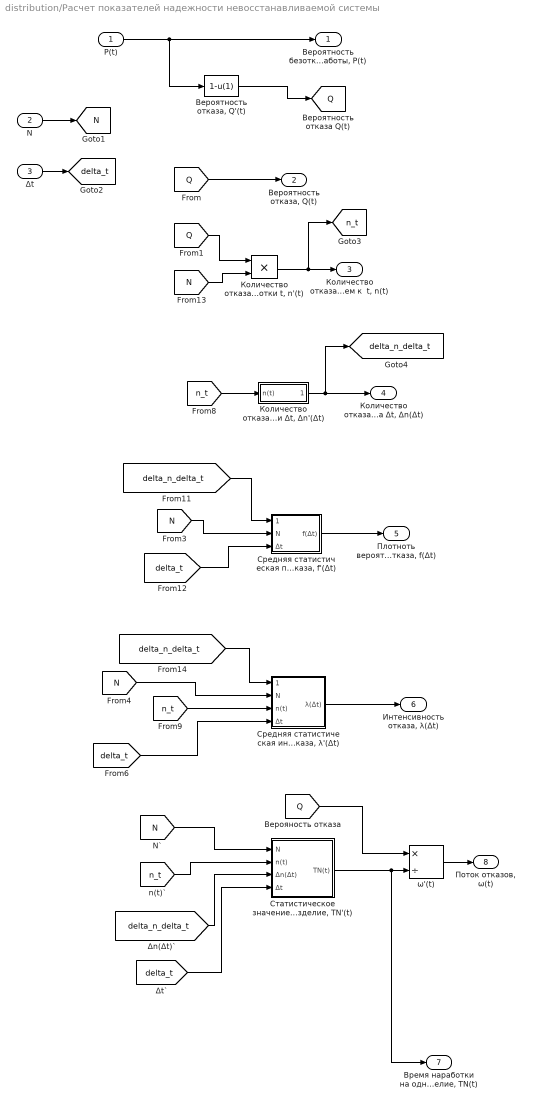
== system distribution/Расчет показателей надежности невосстанавливаемой системы ==
  Р(t) : Inport
  N : Inport  Port=2
  Δt : Inport  Port=3
  ω'(t) : Product  Inputs=*/
  "Вероятность отказа, Q'(t)" : Fcn  Expr=1-u(1)
  "Количество отказавших систем к моменту наработки t, n'(t)" : Product
  "Количество отказавших систем на интервалах наработки Δt, Δn'(Δt)" : Subsystem
  "Средняя статистическая интенсивность отказа, λ'(Δt)" : Subsystem
  "Средняя статистическая плотноть вероятности отказа, f'(Δt)" : Subsystem
  "Статистическое значение среднего времени наработки на одно изделие, TN'(t)" : Subsystem
  "Вероятность безотказной работы, Р(t)" : Outport
  "Вероятность отказа, Q(t)" : Outport  Port=2
  "Количество отказавших систем к  t, n(t)" : Outport  Port=3
  "Количество отказавших систем на Δt, Δn(Δt)" : Outport  Port=4
  "Плотноть вероятности отказа, f(Δt)" : Outport  Port=5
  "Интенсивность отказа, λ(Δt)" : Outport  Port=6
  "Время наработки на одно изделие, TN(t)" : Outport  Port=7
  "Поток отказов, ω(t)" : Outport  Port=8
  tag scope: N=global, Q=global, delta_n_delta_t=global, delta_t=global, n_t=global
  wires:
  [delta_n_delta_t] -> "Статистическое значение среднего времени наработки на одно изделие, TN'(t)"/3(Δn(Δt))
  [delta_n_delta_t] -> "Средняя статистическая интенсивность отказа, λ'(Δt)"/1(Δn(Δt))
  [delta_n_delta_t] -> "Средняя статистическая плотноть вероятности отказа, f'(Δt)"/1(Δn(Δt))
  [N] -> "Количество отказавших систем к моменту наработки t, n'(t)"/2
  [delta_t] -> "Средняя статистическая плотноть вероятности отказа, f'(Δt)"/3(Δt)
  [n_t] -> "Статистическое значение среднего времени наработки на одно изделие, TN'(t)"/2(n(t))
  [n_t] -> "Средняя статистическая интенсивность отказа, λ'(Δt)"/3(n(t))
  [n_t] -> "Количество отказавших систем на интервалах наработки Δt, Δn'(Δt)"/1(n(t))
  [delta_t] -> "Статистическое значение среднего времени наработки на одно изделие, TN'(t)"/4(Δt)
  [delta_t] -> "Средняя статистическая интенсивность отказа, λ'(Δt)"/4(Δt)
  [N] -> "Статистическое значение среднего времени наработки на одно изделие, TN'(t)"/1(N)
  [N] -> "Средняя статистическая интенсивность отказа, λ'(Δt)"/2(N)
  [N] -> "Средняя статистическая плотноть вероятности отказа, f'(Δt)"/2(N)
  [Q] -> ω'(t)/1
  [Q] -> "Количество отказавших систем к моменту наработки t, n'(t)"/1
  [Q] -> "Вероятность отказа, Q(t)"/1
  ω'(t)/1 -> "Поток отказов, ω(t)"/1
  "Вероятность отказа, Q'(t)"/1 -> [Q]
  "Статистическое значение среднего времени наработки на одно изделие, TN'(t)"/1(TN(t)) -> ω'(t)/2, "Время наработки на одно изделие, TN(t)"/1
  N/1 -> [N]
  "Средняя статистическая интенсивность отказа, λ'(Δt)"/1(λ(Δt)) -> "Интенсивность отказа, λ(Δt)"/1
  "Средняя статистическая плотноть вероятности отказа, f'(Δt)"/1(f(Δt)) -> "Плотноть вероятности отказа, f(Δt)"/1
  "Количество отказавших систем к моменту наработки t, n'(t)"/1 -> "Количество отказавших систем к  t, n(t)"/1, [n_t]
  "Количество отказавших систем на интервалах наработки Δt, Δn'(Δt)"/1(Δn(Δt)) -> "Количество отказавших систем на Δt, Δn(Δt)"/1, [delta_n_delta_t]
  Δt/1 -> [delta_t]
  Р(t)/1 -> "Вероятность безотказной работы, Р(t)"/1, "Вероятность отказа, Q'(t)"/1

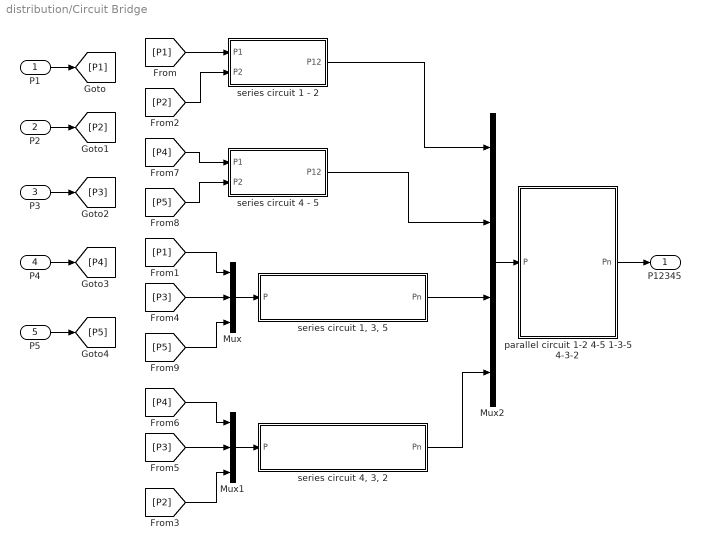
== system distribution/Сircuit Bridge ==
  P1 : Inport
  P2 : Inport  Port=2
  P3 : Inport  Port=3
  P4 : Inport  Port=4
  P5 : Inport  Port=5
  Mux : Mux  Inputs=3
  Mux1 : Mux  Inputs=3
  Mux2 : Mux
  parallel circuit 1-2 4-5 1-3-5 4-3-2 : Subsystem  mask(Сircuit n Parallel){}
      mask help:
      | <p>Возвращает вероятность безотказной работы n параллельно соединенных
      | элементов.</p>
      | <p>В системе с параллельной структурой отказ системы в целом происходит только
      | при отказе всех элементов.</p>
      mask Help:
      | <p>Возвращает вероятность безотказной работы n параллельно соединенных
      | элементов.</p>
      | <p>Входной параметр P - массив вероятностей безотказной работы элементов.</p>
      | <p>Выходной параметр Pт - вероятность безотказной работы n параллельно
      | соединенных элементов.</p>
      mask Display:
      | image('images\png\parallel.png')
      | port_label('input', 1, 'P')
      | port_label('output', 1, 'Pn')
  series circuit 1 - 2 : Subsystem  mask(Сircuit Series){}
      mask help:
      | <p>Возвращает вероятность безотказной работы двух последовательно соединенных
      | элементов.</p>
      | <p>В системе с последовательной структурой отказ любого компонента приводит
      | к отказу системы в целом.</p>
      mask Help:
      | <p>Возвращает вероятность безотказной работы двух последовательно соединенных
      | элементов.</p>
      | <p>Входные параметры:</p>
      | <p>P1 - вероятность безотказной работы первого элемента,</p>
      | <p>P2 - вероятность безотказной работы второго элемента.</p>
      | <p>Выходной параметр P12 - вероятность безотказной работы двух последовательно
      | соединенных элементов.</p>
      mask Display:
      | image('images/png/series2.png')
      | port_label('input', 1, 'P1')
      | port_label('input', 2, 'P2')
      | port_label('output', 1, 'P12')
  "series circuit 1, 3, 5" : Subsystem  mask(Сircuit n Series){}
      mask help:
      | <p>Возвращает вероятность безотказной работы n последовательно соединенных
      | элементов.</p>
      | <p>В системе с последовательной структурой отказ любого компонента приводит
      | к отказу системы в целом.</p>
      mask Help:
      | <p>Возвращает вероятность безотказной работы n последовательно соединенных
      | элементов.</p>
      | <p>Входной параметр P - массив вероятностей безотказной работы n элементов.</p>
      | <p>Выходной параметр Pn - вероятность безотказной работы n последовательно
      | соединенных элементов.</p>
      mask Display:
      | image('images\png\series.png')
      | port_label('input', 1, 'P')
      | port_label('output', 1, 'Pn')
  series circuit 4 - 5 : Subsystem  mask(Сircuit Series){}
      mask help:
      | <p>Возвращает вероятность безотказной работы двух последовательно соединенных
      | элементов.</p>
      | <p>В системе с последовательной структурой отказ любого компонента приводит
      | к отказу системы в целом.</p>
      mask Help:
      | <p>Возвращает вероятность безотказной работы двух последовательно соединенных
      | элементов.</p>
      | <p>Входные параметры:</p>
      | <p>P1 - вероятность безотказной работы первого элемента,</p>
      | <p>P2 - вероятность безотказной работы второго элемента.</p>
      | <p>Выходной параметр P12 - вероятность безотказной работы двух последовательно
      | соединенных элементов.</p>
      mask Display:
      | image('images/png/series2.png')
      | port_label('input', 1, 'P1')
      | port_label('input', 2, 'P2')
      | port_label('output', 1, 'P12')
  "series circuit 4, 3, 2" : Subsystem  mask(Сircuit n Series){}
      mask help:
      | <p>Возвращает вероятность безотказной работы n последовательно соединенных
      | элементов.</p>
      | <p>В системе с последовательной структурой отказ любого компонента приводит
      | к отказу системы в целом.</p>
      mask Help:
      | <p>Возвращает вероятность безотказной работы n последовательно соединенных
      | элементов.</p>
      | <p>Входной параметр P - массив вероятностей безотказной работы n элементов.</p>
      | <p>Выходной параметр Pn - вероятность безотказной работы n последовательно
      | соединенных элементов.</p>
      mask Display:
      | image('images\png\series.png')
      | port_label('input', 1, 'P')
      | port_label('output', 1, 'Pn')
  P12345 : Outport
  wires:
  P1/1 -> [P1]
  [P3] -> Mux1/2
  P5/1 -> [P5]
  [P5] -> Mux/3
  "series circuit 1, 3, 5"/1(Pn) -> Mux2/3
  [P4] -> Mux1/1
  [P3] -> Mux/2
  "series circuit 4, 3, 2"/1(Pn) -> Mux2/4
  P2/1 -> [P2]
  [P5] -> series circuit 4 - 5/2(P2)
  series circuit 1 - 2/1(P12) -> Mux2/1
  [P2] -> series circuit 1 - 2/2(P2)
  P3/1 -> [P3]
  series circuit 4 - 5/1(P12) -> Mux2/2
  parallel circuit 1-2 4-5 1-3-5 4-3-2/1(Pn) -> P12345/1
  [P1] -> Mux/1
  [P4] -> series circuit 4 - 5/1(P1)
  P4/1 -> [P4]
  [P1] -> series circuit 1 - 2/1(P1)
  Mux/1 -> "series circuit 1, 3, 5"/1(P)
  [P2] -> Mux1/3
  Mux1/1 -> "series circuit 4, 3, 2"/1(P)
  Mux2/1 -> parallel circuit 1-2 4-5 1-3-5 4-3-2/1(P)

== system distribution/Сircuit Parallel ==
  P1 : Inport
  P2 : Inport  Port=2
  Fcn1 : Fcn  Expr=1-((1-u(1))*(1-u(2)))
  Mux1 : Mux  Inputs=2
  P12 : Outport
  wires:
  P2/1 -> Mux1/2
  Mux1/1 -> Fcn1/1
  Fcn1/1 -> P12/1
  P1/1 -> Mux1/1

== system distribution/Сircuit Series ==
  note: вероятность безотказной
      | работы первого элемента
  note: вероятность безотказной
      | работы второго элемента
  P1 : Inport
  P2 : Inport  Port=2
  Fcn : Fcn  Expr=u(1)*u(2)
  Mux : Mux  Inputs=2
  P12 : Outport
  wires:
  Mux/1 -> Fcn/1
  P1/1 -> Mux/1
  Fcn/1 -> P12/1
  P2/1 -> Mux/2

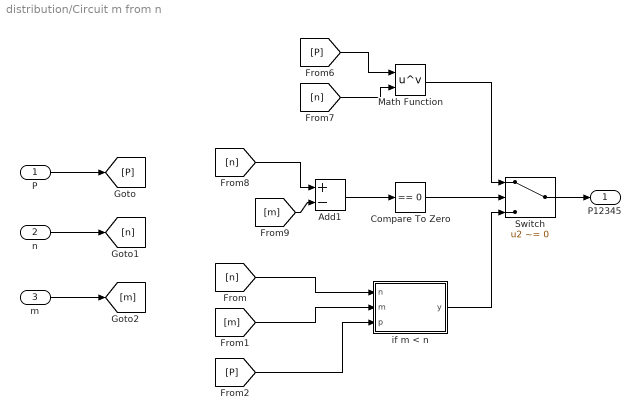
== system distribution/Сircuit m from n ==
  P : Inport
  n : Inport  Port=2
  m : Inport  Port=3
  Add1 : Sum  Inputs=+-
  Compare To Zero : simulink/Logic and Bit Operations/Compare To Zero  relop===  OutDataTypeStr=boolean
  Math Function : Math  Operator=pow  SaturateOnIntegerOverflow=on
  Switch : Switch  Criteria=u2 ~= 0
  if m < n : MATLAB Function  TreatAsAtomicUnit=on
  P12345 : Outport
  wires:
  Math Function/1 -> Switch/1
  n/1 -> [n]
  P/1 -> [P]
  [m] -> Add1/2
  Switch/1 -> P12345/1
  [n] -> Math Function/2
  [m] -> if m < n/2(m)
  [P] -> if m < n/3(p)
  if m < n/1(y) -> Switch/3
  [n] -> if m < n/1(n)
  [n] -> Add1/1
  Compare To Zero/1 -> Switch/2
  [P] -> Math Function/1
  Add1/1 -> Compare To Zero/1
  m/1 -> [m]

== system distribution/Сircuit n Parallel ==
  P : Inport
  n Parallel Function : MATLAB Function  TreatAsAtomicUnit=on
  Pn : Outport
  wires:
  P/1 -> n Parallel Function/1(P)
  n Parallel Function/1(Pn) -> Pn/1

== system distribution/Сircuit n Series ==
  P : Inport
  n Series Function : MATLAB Function  TreatAsAtomicUnit=on
  Pn : Outport
  wires:
  P/1 -> n Series Function/1(P)
  n Series Function/1(Pn) -> Pn/1

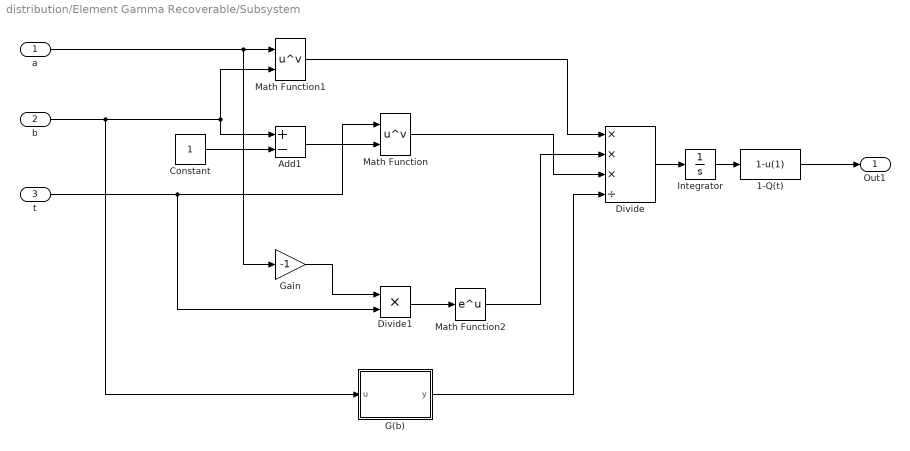
== system distribution/Element Gamma Recoverable/Subsystem ==
  a : Inport
  b : Inport  Port=2
  t : Inport  Port=3
  1-Q(t) : Fcn  Expr=1-u(1)
  Add1 : Sum  Inputs=+-
  Constant : Constant
  Divide : Product  Inputs=***/
  Divide1 : Product  Inputs=**
  G(b) : MATLAB Function  TreatAsAtomicUnit=on
  Gain : Gain  Gain=-1
  Integrator : Integrator
  Math Function : Math  Operator=pow  SaturateOnIntegerOverflow=on
  Math Function1 : Math  Operator=pow  SaturateOnIntegerOverflow=on
  Math Function2 : Math  SaturateOnIntegerOverflow=on
  Out1 : Outport
  wires:
  b/1 -> Math Function1/2, Add1/1, G(b)/1(u)
  Constant/1 -> Add1/2
  a/1 -> Math Function1/1, Gain/1
  Math Function1/1 -> Divide/1
  Divide/1 -> Integrator/1
  Integrator/1 -> 1-Q(t)/1
  Math Function/1 -> Divide/3
  Add1/1 -> Math Function/2
  Gain/1 -> Divide1/1
  Divide1/1 -> Math Function2/1
  Math Function2/1 -> Divide/2
  G(b)/1(y) -> Divide/4
  1-Q(t)/1 -> Out1/1
  t/1 -> Divide1/2, Math Function/1

== system distribution/Расчет показателей надежности невосстанавливаемой системы/Количество отказавших систем на интервалах наработки Δt, Δn'(Δt) ==
  n(t) : Inport
  Display1 : Display
  Display2 : Display
  Display3 : Display
  Fcn : Fcn  Expr=u(1)-u(2)
  Memory : Memory
  Mux : Mux  Inputs=2
  Δn(Δt) : Outport
  wires:
  Memory/1 -> Mux/2, Display3/1
  n(t)/1 -> Mux/1, Memory/1, Display2/1
  Mux/1 -> Fcn/1
  Fcn/1 -> Δn(Δt)/1, Display1/1

== system distribution/Расчет показателей надежности невосстанавливаемой системы/Средняя статистическая интенсивность отказа, λ'(Δt) ==
  Δn(Δt) : Inport
  N : Inport  Port=2
  n(t) : Inport  Port=3
  Δt : Inport  Port=4
  Add : Sum  Inputs=+-+
  Divide : Product  Inputs=**
  Divide1 : Product  Inputs=*/
  Gain : Gain  Gain=0.5
  λ(Δt) : Outport
  wires:
  Δn(Δt)/1 -> Divide1/1, Gain/1
  Add/1 -> Divide/1
  Gain/1 -> Add/3
  Divide/1 -> Divide1/2
  Δt/1 -> Divide/2
  N/1 -> Add/1
  n(t)/1 -> Add/2
  Divide1/1 -> λ(Δt)/1

== system distribution/Расчет показателей надежности невосстанавливаемой системы/Средняя статистическая плотноть вероятности отказа, f'(Δt) ==
  Δn(Δt) : Inport
  N : Inport  Port=2
  Δt : Inport  Port=3
  Divide : Product  Inputs=**
  Divide1 : Product  Inputs=*/
  f(Δt) : Outport
  wires:
  N/1 -> Divide/1
  Δn(Δt)/1 -> Divide1/1
  Divide/1 -> Divide1/2
  Divide1/1 -> f(Δt)/1
  Δt/1 -> Divide/2

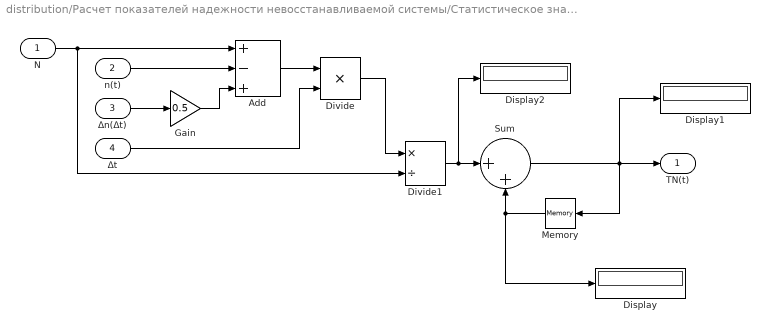
== system distribution/Расчет показателей надежности невосстанавливаемой системы/Статистическое значение среднего времени наработки на одно изделие, TN'(t) ==
  N : Inport
  n(t) : Inport  Port=2
  Δn(Δt) : Inport  Port=3
  Δt : Inport  Port=4
  Add : Sum  Inputs=+-+
  Display : Display
  Display1 : Display
  Display2 : Display
  Divide : Product  Inputs=**
  Divide1 : Product  Inputs=*/
  Gain : Gain  Gain=0.5
  Memory : Memory
  Sum : Sum  Inputs=|++
  TN(t) : Outport
  wires:
  Memory/1 -> Sum/2, Display/1
  Sum/1 -> TN(t)/1, Memory/1, Display1/1
  Δt/1 -> Divide/2
  N/1 -> Add/1, Divide1/2
  Δn(Δt)/1 -> Gain/1
  n(t)/1 -> Add/2
  Divide/1 -> Divide1/1
  Gain/1 -> Add/3
  Add/1 -> Divide/1
  Divide1/1 -> Sum/1, Display2/1

== system distribution/Сircuit Bridge/parallel circuit 1-2 4-5 1-3-5 4-3-2 ==
  P : Inport
  n Parallel Function : MATLAB Function  TreatAsAtomicUnit=on
  Pn : Outport
  wires:
  P/1 -> n Parallel Function/1(P)
  n Parallel Function/1(Pn) -> Pn/1

== system distribution/Сircuit Bridge/series circuit 1 - 2 ==
  P1 : Inport
  P2 : Inport  Port=2
  Fcn : Fcn  Expr=u(1)*u(2)
  Mux : Mux  Inputs=2
  P12 : Outport
  wires:
  Mux/1 -> Fcn/1
  P1/1 -> Mux/1
  Fcn/1 -> P12/1
  P2/1 -> Mux/2

== system distribution/Сircuit Bridge/series circuit 1, 3, 5 ==
  P : Inport
  n Series Function : MATLAB Function  TreatAsAtomicUnit=on
  Pn : Outport
  wires:
  P/1 -> n Series Function/1(P)
  n Series Function/1(Pn) -> Pn/1

== system distribution/Сircuit Bridge/series circuit 4 - 5 ==
  P1 : Inport
  P2 : Inport  Port=2
  Fcn : Fcn  Expr=u(1)*u(2)
  Mux : Mux  Inputs=2
  P12 : Outport
  wires:
  Mux/1 -> Fcn/1
  P1/1 -> Mux/1
  Fcn/1 -> P12/1
  P2/1 -> Mux/2

== system distribution/Сircuit Bridge/series circuit 4, 3, 2 ==
  P : Inport
  n Series Function : MATLAB Function  TreatAsAtomicUnit=on
  Pn : Outport
  wires:
  P/1 -> n Series Function/1(P)
  n Series Function/1(Pn) -> Pn/1

== matlab function distribution/Сircuit n Parallel/n Parallel Function ==
  data: Pn output; P input
function Pn = fcn(P)
[n,col]=size(P);
u=1;
for i=1:n
   u=u*(1-P(i)); 
end
Pn = 1 - u;

== matlab function distribution/Сircuit n Series/n Series Function ==
  data: Pn output; P input
function Pn = fcn(P)
[n,col]=size(P);
u=1;
for i=1:n
   u=u*P(i); 
end
Pn = u;

== matlab function distribution/Сircuit Bridge/series circuit 1, 3, 5/n Series Function ==
  data: Pn output; P input
function Pn = fcn(P)
[n,col]=size(P);
u=1;
for i=1:n
   u=u*P(i); 
end

Pn = u;

== matlab function distribution/Сircuit Bridge/series circuit 4, 3, 2/n Series Function ==
  data: Pn output; P input
function Pn = fcn(P)
[n,col]=size(P);
u=1;
for i=1:n
   u=u*P(i); 
end

Pn = u;

== matlab function distribution/Сircuit Bridge/parallel circuit 1-2 4-5 1-3-5 4-3-2/n Parallel Function ==
  data: Pn output; P input
function Pn = fcn(P)
[n,col]=size(P);
u=1;
for i=1:n
   u=u*(1-P(i)); 
end

Pn = 1 - u;

== matlab function distribution/Сircuit m from n/if m < n ==
  data: n input; y output; m input; p input
function y = fcn(n,m,p)
Pn = 0;
q = 1-p;
for i=m:n
    k = n-i;
Pn = Pn + (factorial(n)/(factorial(i)*factorial(k)))*power(p,i)*power(q,k);
end
y=Pn;

== matlab function distribution/Element Gamma/G(b) ==
  data: u input; y output
function y = fcn(u)
%#codegen
y = gamma(u);

== matlab function distribution/Element Normal/MATLAB Function ==
  data: t input; y output; sigma input; M input
function y = fcn(t,sigma,M)
y=normcdf((t-M)/sigma);

== matlab function distribution/Element Lognormal /MATLAB Function ==
  data: t input; y output; sigma input; M input
function y = fcn(t,sigma,M)
y=normcdf((log(t)-M)/sigma);

== stateflow chart distribution/Element Weibull Recoverable/Chart ==
  state start
    entry: delta_P=dP;
    t_z=0;
    P=P0;
    t0=0;
    i=0;
  state first_sec
    entry:t0=t; i=i+1;dt=t;
    during:P=0;
  state second
    entry:
    tv=t-t0;
    P=P0-dP*i;
    during:tv=t-t0;
    P=P0-dP*i;
  state first
    during: tv=t-t0;
    P=P0-dP*i;
  state third
    entry: t0=t;
    during:P=P0-dP*i;
  (default) -> start
  first -> first_sec : [P<=Pz]
  first_sec -> second : [t-dt>=delta_t]
  start -> first : [t~=0]
  second -> first [order 2] : [P>Pz]
  second -> third [order 1] : [P0==1 && P<=Pz]
  data: dP input; t input; Pz input; delta_P local; t_z local; tv output; P output; i local; t0 local; P0 input; delta_t input; dt local
